simulink model "Meccanum_drive"  (R2025b)
settings: Solver=ode45  StartTime=0.0  StopTime=sim_stop_time  FixedStep=0.001  MaxStep=sim_step_time  RelTol=1e-8  AbsTol=1e-8
undefined symbols (not defined in the file): Bm, Jm, K, Lm, Rm, sim_step_time, vref
settings Model: Creator=shashi  LastModifiedBy=shashi
settings SolverCC: AutoScaleAbsTol=off
settings DataIOCC: SaveOutput=off  SignalLogging=off  DSMLogging=off  SaveTime=off  ReturnWorkspaceOutputs=off

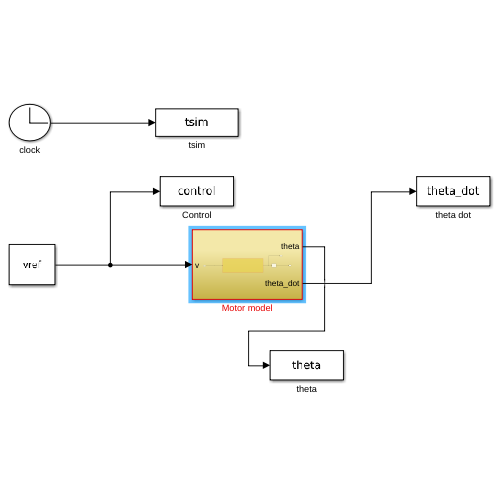
[thumbnail: Simulink's stored preview of the top-level diagram]
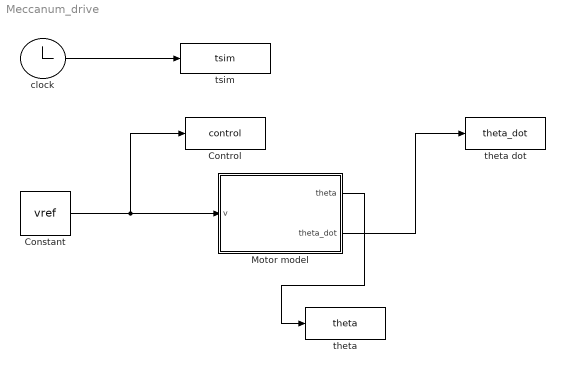
== system Meccanum_drive ==
  Constant : Constant  Value=vref  SampleTime=sim_step_time
  Control : ToWorkspace  VariableName=control  SampleTime=sim_step_time
      settings: Save2DSignal=2-D array (concatenate along first dimension)
  Motor model : Subsystem
  clock : Clock
  theta : ToWorkspace  VariableName=theta  SampleTime=sim_step_time
  theta dot : ToWorkspace  VariableName=theta_dot  SampleTime=sim_step_time
      settings: Save2DSignal=2-D array (concatenate along first dimension)
  tsim : ToWorkspace  VariableName=tsim  SampleTime=sim_step_time
      settings: Save2DSignal=2-D array (concatenate along first dimension)
  wires:
  clock/1 -> tsim/1
  Constant/1 -> Motor model/1(v), Control/1
  Motor model/1(theta) -> theta/1
  Motor model/2(theta_dot) -> theta dot/1

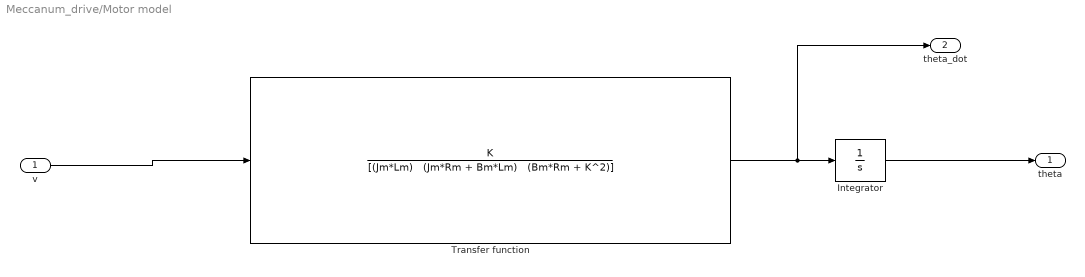
== system Meccanum_drive/Motor model ==
  v : Inport
  Integrator : Integrator
  Transfer function : TransferFcn  Numerator=K  Denominator="[(Jm*Lm)   (Jm*Rm + Bm*Lm)   (Bm*Rm + K^2)]"
  theta : Outport
  theta_dot : Outport  Port=2
  wires:
  v/1 -> Transfer function/1
  Transfer function/1 -> theta_dot/1, Integrator/1
  Integrator/1 -> theta/1
